simulink model "bici_v2"  (R2013a)
settings: Solver=ode3  SolverMode=SingleTasking  StartTime=0.0  StopTime=10.0  RelTol=1e-3
PreLoadFcn:
  | waijung.modelPreload; % Required for working with Waijung Blockset. Do not remove.
undefined symbols (not defined in the file or in its folder): HSEOSC, Link, LQFP176, ST, STM32F417IG
libraries: simulink x6, stm32f4_tim_lib x6, stm32f4_io_lib x2, stm32f4_adc_lib x1, stm32f4_device_config_lib x1
(part 2 of 2)

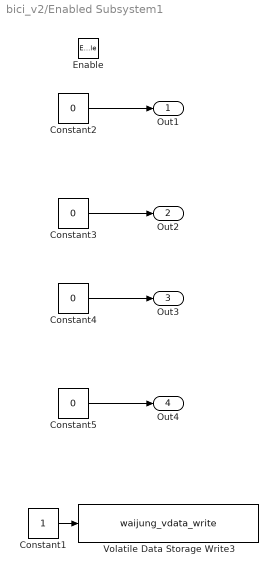
== system bici_v2/Enabled Subsystem1 ==
  Enable : EnablePort
  Constant1 : Constant
  Constant{2..5} (4 alike) : Constant  Value=0
  Volatile Data Storage Write3 : S-Function  FunctionName=waijung_vdata_write  Parameters=storagename,varname,sampletime,sampletimestr,blockid,storagetype,storagetypestr  EnableBusSupport=off  mask(waijung_vdata_write){storagename=c, varname=VolatileDataStorage3_c, sampletime=-1, sampletimestr=0.01, blockid=EnabledSubsystem1VolatileDataStorageWrite3, storagetype=double, storagetypestr=double}
      mask prompts: storagename "Storage Name"; varname "Variable name"; sampletime "Sample time (sec)"; sampletimestr "Compiled sample time (sec) in string"; storagetype "Data type"; storagetypestr "Data type string"
      mask help: This block implements write data to a buffer.
      mask init:
      | waijung_vdata_write_callback('init');
      mask Help: web(fullfile(waijungdocroot,'Volatile_Data_Storage_Write.htm'))
      mask TypeOptions storagename: condicion | c
      mask Callback storagename: waijung_vdata_write_callback('storagename');
      mask Callback varname: waijung_vdata_write_callback('varname');
      mask Callback sampletime: waijung_vdata_write_callback('sampletime');
      mask Callback sampletimestr: waijung_vdata_write_callback('sampletimestr');
      mask Callback blockid: waijung_vdata_write_callback('blockid');
      mask Callback storagetype: waijung_vdata_write_callback('storagetype');
      mask Display: text(0.95, 0.5, 'Buffer: c','ver','middle','hor','right');port_label('input',1,'D1(double)')
  Out1 : Outport
  Out2 : Outport  Port=2
  Out3 : Outport  Port=3
  Out4 : Outport  Port=4
  wires:
  Constant2/1 -> Out1/1
  Constant3/1 -> Out2/1
  Constant1/1 -> Volatile Data Storage Write3/1
  Constant4/1 -> Out3/1
  Constant5/1 -> Out4/1

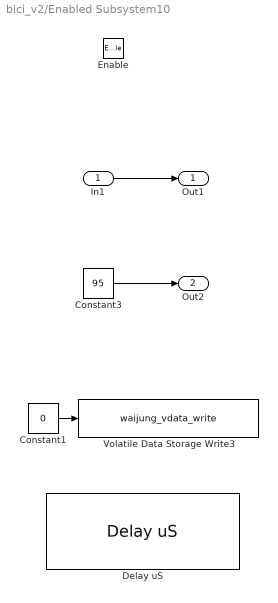
== system bici_v2/Enabled Subsystem10 ==
  In1 : Inport
  Enable : EnablePort
  Constant1 : Constant  Value=0
  Constant3 : Constant  Value=95
  Delay uS : stm32f4_tim_lib/Delay uS  delaytime=1  enableinput=off  enableoutput=off  inputtypearray=[0]  outputtypearray=[0]  sampletime=-1  sampletimestr=0.01  blockid=EnabledSubsystem10DelayuS
  Volatile Data Storage Write3 : S-Function  FunctionName=waijung_vdata_write  Parameters=storagename,varname,sampletime,sampletimestr,blockid,storagetype,storagetypestr  EnableBusSupport=off  mask(waijung_vdata_write){storagename=c, varname=VolatileDataStorage3_c, sampletime=-1, sampletimestr=0.01, blockid=EnabledSubsystem10VolatileDataStorageWrite3, storagetype=double, storagetypestr=double}
      mask prompts: storagename "Storage Name"; varname "Variable name"; sampletime "Sample time (sec)"; sampletimestr "Compiled sample time (sec) in string"; storagetype "Data type"; storagetypestr "Data type string"
      mask help: This block implements write data to a buffer.
      mask init:
      | waijung_vdata_write_callback('init');
      mask Help: web(fullfile(waijungdocroot,'Volatile_Data_Storage_Write.htm'))
      mask TypeOptions storagename: condicion | c
      mask Callback storagename: waijung_vdata_write_callback('storagename');
      mask Callback varname: waijung_vdata_write_callback('varname');
      mask Callback sampletime: waijung_vdata_write_callback('sampletime');
      mask Callback sampletimestr: waijung_vdata_write_callback('sampletimestr');
      mask Callback blockid: waijung_vdata_write_callback('blockid');
      mask Callback storagetype: waijung_vdata_write_callback('storagetype');
      mask Display: text(0.95, 0.5, 'Buffer: c','ver','middle','hor','right');port_label('input',1,'D1(double)')
  Out1 : Outport
  Out2 : Outport  Port=2
  wires:
  Constant3/1 -> Out2/1
  Constant1/1 -> Volatile Data Storage Write3/1
  In1/1 -> Out1/1

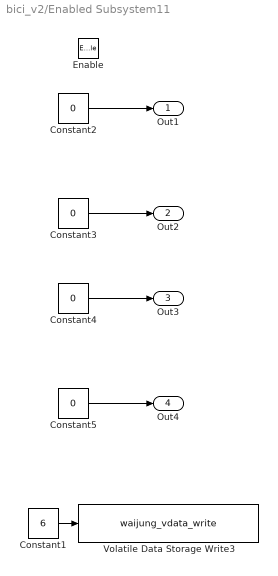
== system bici_v2/Enabled Subsystem11 ==
  Enable : EnablePort
  Constant1 : Constant  Value=6
  Constant{2..5} (4 alike) : Constant  Value=0
  Volatile Data Storage Write3 : S-Function  FunctionName=waijung_vdata_write  Parameters=storagename,varname,sampletime,sampletimestr,blockid,storagetype,storagetypestr  EnableBusSupport=off  mask(waijung_vdata_write){storagename=c, varname=VolatileDataStorage3_c, sampletime=-1, sampletimestr=0.01, blockid=EnabledSubsystem11VolatileDataStorageWrite3, storagetype=double, storagetypestr=double}
      mask prompts: storagename "Storage Name"; varname "Variable name"; sampletime "Sample time (sec)"; sampletimestr "Compiled sample time (sec) in string"; storagetype "Data type"; storagetypestr "Data type string"
      mask help: This block implements write data to a buffer.
      mask init:
      | waijung_vdata_write_callback('init');
      mask Help: web(fullfile(waijungdocroot,'Volatile_Data_Storage_Write.htm'))
      mask TypeOptions storagename: condicion | c
      mask Callback storagename: waijung_vdata_write_callback('storagename');
      mask Callback varname: waijung_vdata_write_callback('varname');
      mask Callback sampletime: waijung_vdata_write_callback('sampletime');
      mask Callback sampletimestr: waijung_vdata_write_callback('sampletimestr');
      mask Callback blockid: waijung_vdata_write_callback('blockid');
      mask Callback storagetype: waijung_vdata_write_callback('storagetype');
      mask Display: text(0.95, 0.5, 'Buffer: c','ver','middle','hor','right');port_label('input',1,'D1(double)')
  Out1 : Outport
  Out2 : Outport  Port=2
  Out3 : Outport  Port=3
  Out4 : Outport  Port=4
  wires:
  Constant2/1 -> Out1/1
  Constant3/1 -> Out2/1
  Constant1/1 -> Volatile Data Storage Write3/1
  Constant4/1 -> Out3/1
  Constant5/1 -> Out4/1

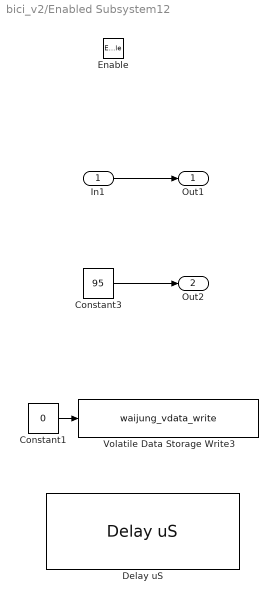
== system bici_v2/Enabled Subsystem12 ==
  In1 : Inport
  Enable : EnablePort
  Constant1 : Constant  Value=0
  Constant3 : Constant  Value=95
  Delay uS : stm32f4_tim_lib/Delay uS  delaytime=1  enableinput=off  enableoutput=off  inputtypearray=[0]  outputtypearray=[0]  sampletime=-1  sampletimestr=0.01  blockid=EnabledSubsystem12DelayuS
  Volatile Data Storage Write3 : S-Function  FunctionName=waijung_vdata_write  Parameters=storagename,varname,sampletime,sampletimestr,blockid,storagetype,storagetypestr  EnableBusSupport=off  mask(waijung_vdata_write){storagename=c, varname=VolatileDataStorage3_c, sampletime=-1, sampletimestr=0.01, blockid=EnabledSubsystem12VolatileDataStorageWrite3, storagetype=double, storagetypestr=double}
      mask prompts: storagename "Storage Name"; varname "Variable name"; sampletime "Sample time (sec)"; sampletimestr "Compiled sample time (sec) in string"; storagetype "Data type"; storagetypestr "Data type string"
      mask help: This block implements write data to a buffer.
      mask init:
      | waijung_vdata_write_callback('init');
      mask Help: web(fullfile(waijungdocroot,'Volatile_Data_Storage_Write.htm'))
      mask TypeOptions storagename: condicion | c
      mask Callback storagename: waijung_vdata_write_callback('storagename');
      mask Callback varname: waijung_vdata_write_callback('varname');
      mask Callback sampletime: waijung_vdata_write_callback('sampletime');
      mask Callback sampletimestr: waijung_vdata_write_callback('sampletimestr');
      mask Callback blockid: waijung_vdata_write_callback('blockid');
      mask Callback storagetype: waijung_vdata_write_callback('storagetype');
      mask Display: text(0.95, 0.5, 'Buffer: c','ver','middle','hor','right');port_label('input',1,'D1(double)')
  Out1 : Outport
  Out2 : Outport  Port=2
  wires:
  Constant3/1 -> Out2/1
  Constant1/1 -> Volatile Data Storage Write3/1
  In1/1 -> Out1/1

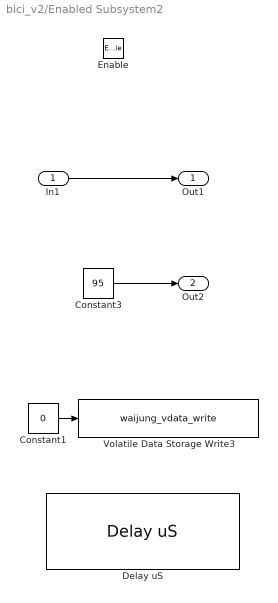
== system bici_v2/Enabled Subsystem2 ==
  In1 : Inport
  Enable : EnablePort
  Constant1 : Constant  Value=0
  Constant3 : Constant  Value=95
  Delay uS : stm32f4_tim_lib/Delay uS  delaytime=1  enableinput=off  enableoutput=off  inputtypearray=[0]  outputtypearray=[0]  sampletime=-1  sampletimestr=0.01  blockid=EnabledSubsystem2DelayuS
  Volatile Data Storage Write3 : S-Function  FunctionName=waijung_vdata_write  Parameters=storagename,varname,sampletime,sampletimestr,blockid,storagetype,storagetypestr  EnableBusSupport=off  mask(waijung_vdata_write){storagename=c, varname=VolatileDataStorage3_c, sampletime=-1, sampletimestr=0.01, blockid=EnabledSubsystem2VolatileDataStorageWrite3, storagetype=double, storagetypestr=double}
      mask prompts: storagename "Storage Name"; varname "Variable name"; sampletime "Sample time (sec)"; sampletimestr "Compiled sample time (sec) in string"; storagetype "Data type"; storagetypestr "Data type string"
      mask help: This block implements write data to a buffer.
      mask init:
      | waijung_vdata_write_callback('init');
      mask Help: web(fullfile(waijungdocroot,'Volatile_Data_Storage_Write.htm'))
      mask TypeOptions storagename: condicion | c
      mask Callback storagename: waijung_vdata_write_callback('storagename');
      mask Callback varname: waijung_vdata_write_callback('varname');
      mask Callback sampletime: waijung_vdata_write_callback('sampletime');
      mask Callback sampletimestr: waijung_vdata_write_callback('sampletimestr');
      mask Callback blockid: waijung_vdata_write_callback('blockid');
      mask Callback storagetype: waijung_vdata_write_callback('storagetype');
      mask Display: text(0.95, 0.5, 'Buffer: c','ver','middle','hor','right');port_label('input',1,'D1(double)')
  Out1 : Outport
  Out2 : Outport  Port=2
  wires:
  Constant3/1 -> Out2/1
  Constant1/1 -> Volatile Data Storage Write3/1
  In1/1 -> Out1/1

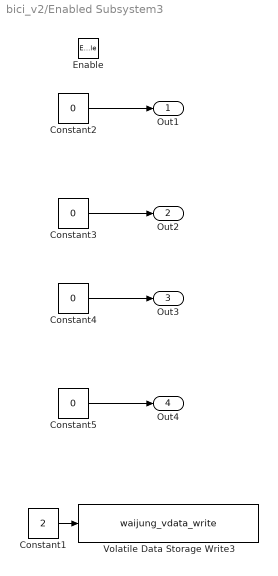
== system bici_v2/Enabled Subsystem3 ==
  Enable : EnablePort
  Constant1 : Constant  Value=2
  Constant{2..5} (4 alike) : Constant  Value=0
  Volatile Data Storage Write3 : S-Function  FunctionName=waijung_vdata_write  Parameters=storagename,varname,sampletime,sampletimestr,blockid,storagetype,storagetypestr  EnableBusSupport=off  mask(waijung_vdata_write){storagename=c, varname=VolatileDataStorage3_c, sampletime=-1, sampletimestr=0.01, blockid=EnabledSubsystem3VolatileDataStorageWrite3, storagetype=double, storagetypestr=double}
      mask prompts: storagename "Storage Name"; varname "Variable name"; sampletime "Sample time (sec)"; sampletimestr "Compiled sample time (sec) in string"; storagetype "Data type"; storagetypestr "Data type string"
      mask help: This block implements write data to a buffer.
      mask init:
      | waijung_vdata_write_callback('init');
      mask Help: web(fullfile(waijungdocroot,'Volatile_Data_Storage_Write.htm'))
      mask TypeOptions storagename: condicion | c
      mask Callback storagename: waijung_vdata_write_callback('storagename');
      mask Callback varname: waijung_vdata_write_callback('varname');
      mask Callback sampletime: waijung_vdata_write_callback('sampletime');
      mask Callback sampletimestr: waijung_vdata_write_callback('sampletimestr');
      mask Callback blockid: waijung_vdata_write_callback('blockid');
      mask Callback storagetype: waijung_vdata_write_callback('storagetype');
      mask Display: text(0.95, 0.5, 'Buffer: c','ver','middle','hor','right');port_label('input',1,'D1(double)')
  Out1 : Outport
  Out2 : Outport  Port=2
  Out3 : Outport  Port=3
  Out4 : Outport  Port=4
  wires:
  Constant2/1 -> Out1/1
  Constant3/1 -> Out2/1
  Constant1/1 -> Volatile Data Storage Write3/1
  Constant4/1 -> Out3/1
  Constant5/1 -> Out4/1

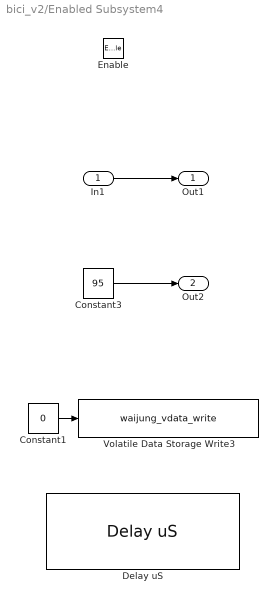
== system bici_v2/Enabled Subsystem4 ==
  In1 : Inport
  Enable : EnablePort
  Constant1 : Constant  Value=0
  Constant3 : Constant  Value=95
  Delay uS : stm32f4_tim_lib/Delay uS  delaytime=1  enableinput=off  enableoutput=off  inputtypearray=[0]  outputtypearray=[0]  sampletime=-1  sampletimestr=0.01  blockid=EnabledSubsystem4DelayuS
  Volatile Data Storage Write3 : S-Function  FunctionName=waijung_vdata_write  Parameters=storagename,varname,sampletime,sampletimestr,blockid,storagetype,storagetypestr  EnableBusSupport=off  mask(waijung_vdata_write){storagename=c, varname=VolatileDataStorage3_c, sampletime=-1, sampletimestr=0.01, blockid=EnabledSubsystem4VolatileDataStorageWrite3, storagetype=double, storagetypestr=double}
      mask prompts: storagename "Storage Name"; varname "Variable name"; sampletime "Sample time (sec)"; sampletimestr "Compiled sample time (sec) in string"; storagetype "Data type"; storagetypestr "Data type string"
      mask help: This block implements write data to a buffer.
      mask init:
      | waijung_vdata_write_callback('init');
      mask Help: web(fullfile(waijungdocroot,'Volatile_Data_Storage_Write.htm'))
      mask TypeOptions storagename: condicion | c
      mask Callback storagename: waijung_vdata_write_callback('storagename');
      mask Callback varname: waijung_vdata_write_callback('varname');
      mask Callback sampletime: waijung_vdata_write_callback('sampletime');
      mask Callback sampletimestr: waijung_vdata_write_callback('sampletimestr');
      mask Callback blockid: waijung_vdata_write_callback('blockid');
      mask Callback storagetype: waijung_vdata_write_callback('storagetype');
      mask Display: text(0.95, 0.5, 'Buffer: c','ver','middle','hor','right');port_label('input',1,'D1(double)')
  Out1 : Outport
  Out2 : Outport  Port=2
  wires:
  Constant3/1 -> Out2/1
  Constant1/1 -> Volatile Data Storage Write3/1
  In1/1 -> Out1/1

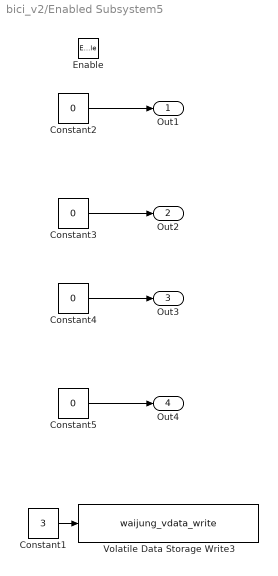
== system bici_v2/Enabled Subsystem5 ==
  Enable : EnablePort
  Constant1 : Constant  Value=3
  Constant{2..5} (4 alike) : Constant  Value=0
  Volatile Data Storage Write3 : S-Function  FunctionName=waijung_vdata_write  Parameters=storagename,varname,sampletime,sampletimestr,blockid,storagetype,storagetypestr  EnableBusSupport=off  mask(waijung_vdata_write){storagename=c, varname=VolatileDataStorage3_c, sampletime=-1, sampletimestr=0.01, blockid=EnabledSubsystem5VolatileDataStorageWrite3, storagetype=double, storagetypestr=double}
      mask prompts: storagename "Storage Name"; varname "Variable name"; sampletime "Sample time (sec)"; sampletimestr "Compiled sample time (sec) in string"; storagetype "Data type"; storagetypestr "Data type string"
      mask help: This block implements write data to a buffer.
      mask init:
      | waijung_vdata_write_callback('init');
      mask Help: web(fullfile(waijungdocroot,'Volatile_Data_Storage_Write.htm'))
      mask TypeOptions storagename: condicion | c
      mask Callback storagename: waijung_vdata_write_callback('storagename');
      mask Callback varname: waijung_vdata_write_callback('varname');
      mask Callback sampletime: waijung_vdata_write_callback('sampletime');
      mask Callback sampletimestr: waijung_vdata_write_callback('sampletimestr');
      mask Callback blockid: waijung_vdata_write_callback('blockid');
      mask Callback storagetype: waijung_vdata_write_callback('storagetype');
      mask Display: text(0.95, 0.5, 'Buffer: c','ver','middle','hor','right');port_label('input',1,'D1(double)')
  Out1 : Outport
  Out2 : Outport  Port=2
  Out3 : Outport  Port=3
  Out4 : Outport  Port=4
  wires:
  Constant2/1 -> Out1/1
  Constant3/1 -> Out2/1
  Constant1/1 -> Volatile Data Storage Write3/1
  Constant4/1 -> Out3/1
  Constant5/1 -> Out4/1

== system bici_v2/Enabled Subsystem6 ==
  In1 : Inport
  Enable : EnablePort
  Constant1 : Constant  Value=0
  Constant3 : Constant  Value=95
  Delay uS : stm32f4_tim_lib/Delay uS  delaytime=1  enableinput=off  enableoutput=off  inputtypearray=[0]  outputtypearray=[0]  sampletime=-1  sampletimestr=0.01  blockid=EnabledSubsystem6DelayuS
  Volatile Data Storage Write3 : S-Function  FunctionName=waijung_vdata_write  Parameters=storagename,varname,sampletime,sampletimestr,blockid,storagetype,storagetypestr  EnableBusSupport=off  mask(waijung_vdata_write){storagename=c, varname=VolatileDataStorage3_c, sampletime=-1, sampletimestr=0.01, blockid=EnabledSubsystem6VolatileDataStorageWrite3, storagetype=double, storagetypestr=double}
      mask prompts: storagename "Storage Name"; varname "Variable name"; sampletime "Sample time (sec)"; sampletimestr "Compiled sample time (sec) in string"; storagetype "Data type"; storagetypestr "Data type string"
      mask help: This block implements write data to a buffer.
      mask init:
      | waijung_vdata_write_callback('init');
      mask Help: web(fullfile(waijungdocroot,'Volatile_Data_Storage_Write.htm'))
      mask TypeOptions storagename: condicion | c
      mask Callback storagename: waijung_vdata_write_callback('storagename');
      mask Callback varname: waijung_vdata_write_callback('varname');
      mask Callback sampletime: waijung_vdata_write_callback('sampletime');
      mask Callback sampletimestr: waijung_vdata_write_callback('sampletimestr');
      mask Callback blockid: waijung_vdata_write_callback('blockid');
      mask Callback storagetype: waijung_vdata_write_callback('storagetype');
      mask Display: text(0.95, 0.5, 'Buffer: c','ver','middle','hor','right');port_label('input',1,'D1(double)')
  Out1 : Outport
  Out2 : Outport  Port=2
  wires:
  Constant3/1 -> Out2/1
  Constant1/1 -> Volatile Data Storage Write3/1
  In1/1 -> Out1/1

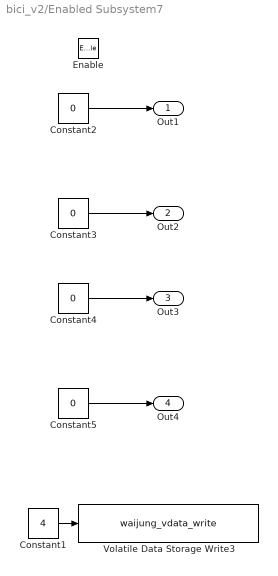
== system bici_v2/Enabled Subsystem7 ==
  Enable : EnablePort
  Constant1 : Constant  Value=4
  Constant{2..5} (4 alike) : Constant  Value=0
  Volatile Data Storage Write3 : S-Function  FunctionName=waijung_vdata_write  Parameters=storagename,varname,sampletime,sampletimestr,blockid,storagetype,storagetypestr  EnableBusSupport=off  mask(waijung_vdata_write){storagename=c, varname=VolatileDataStorage3_c, sampletime=-1, sampletimestr=0.01, blockid=EnabledSubsystem7VolatileDataStorageWrite3, storagetype=double, storagetypestr=double}
      mask prompts: storagename "Storage Name"; varname "Variable name"; sampletime "Sample time (sec)"; sampletimestr "Compiled sample time (sec) in string"; storagetype "Data type"; storagetypestr "Data type string"
      mask help: This block implements write data to a buffer.
      mask init:
      | waijung_vdata_write_callback('init');
      mask Help: web(fullfile(waijungdocroot,'Volatile_Data_Storage_Write.htm'))
      mask TypeOptions storagename: condicion | c
      mask Callback storagename: waijung_vdata_write_callback('storagename');
      mask Callback varname: waijung_vdata_write_callback('varname');
      mask Callback sampletime: waijung_vdata_write_callback('sampletime');
      mask Callback sampletimestr: waijung_vdata_write_callback('sampletimestr');
      mask Callback blockid: waijung_vdata_write_callback('blockid');
      mask Callback storagetype: waijung_vdata_write_callback('storagetype');
      mask Display: text(0.95, 0.5, 'Buffer: c','ver','middle','hor','right');port_label('input',1,'D1(double)')
  Out1 : Outport
  Out2 : Outport  Port=2
  Out3 : Outport  Port=3
  Out4 : Outport  Port=4
  wires:
  Constant2/1 -> Out1/1
  Constant3/1 -> Out2/1
  Constant1/1 -> Volatile Data Storage Write3/1
  Constant4/1 -> Out3/1
  Constant5/1 -> Out4/1

== system bici_v2/Enabled Subsystem8 ==
  In1 : Inport
  Enable : EnablePort
  Constant1 : Constant  Value=0
  Constant3 : Constant  Value=95
  Delay uS : stm32f4_tim_lib/Delay uS  delaytime=1  enableinput=off  enableoutput=off  inputtypearray=[0]  outputtypearray=[0]  sampletime=-1  sampletimestr=0.01  blockid=EnabledSubsystem8DelayuS
  Volatile Data Storage Write3 : S-Function  FunctionName=waijung_vdata_write  Parameters=storagename,varname,sampletime,sampletimestr,blockid,storagetype,storagetypestr  EnableBusSupport=off  mask(waijung_vdata_write){storagename=c, varname=VolatileDataStorage3_c, sampletime=-1, sampletimestr=0.01, blockid=EnabledSubsystem8VolatileDataStorageWrite3, storagetype=double, storagetypestr=double}
      mask prompts: storagename "Storage Name"; varname "Variable name"; sampletime "Sample time (sec)"; sampletimestr "Compiled sample time (sec) in string"; storagetype "Data type"; storagetypestr "Data type string"
      mask help: This block implements write data to a buffer.
      mask init:
      | waijung_vdata_write_callback('init');
      mask Help: web(fullfile(waijungdocroot,'Volatile_Data_Storage_Write.htm'))
      mask TypeOptions storagename: condicion | c
      mask Callback storagename: waijung_vdata_write_callback('storagename');
      mask Callback varname: waijung_vdata_write_callback('varname');
      mask Callback sampletime: waijung_vdata_write_callback('sampletime');
      mask Callback sampletimestr: waijung_vdata_write_callback('sampletimestr');
      mask Callback blockid: waijung_vdata_write_callback('blockid');
      mask Callback storagetype: waijung_vdata_write_callback('storagetype');
      mask Display: text(0.95, 0.5, 'Buffer: c','ver','middle','hor','right');port_label('input',1,'D1(double)')
  Out1 : Outport
  Out2 : Outport  Port=2
  wires:
  Constant3/1 -> Out2/1
  Constant1/1 -> Volatile Data Storage Write3/1
  In1/1 -> Out1/1

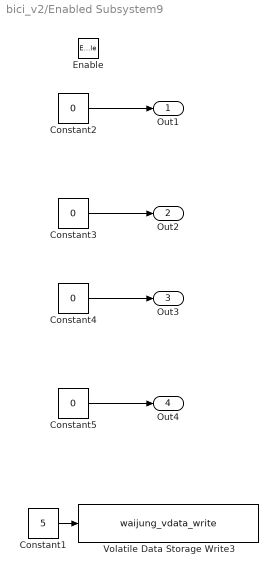
== system bici_v2/Enabled Subsystem9 ==
  Enable : EnablePort
  Constant1 : Constant  Value=5
  Constant{2..5} (4 alike) : Constant  Value=0
  Volatile Data Storage Write3 : S-Function  FunctionName=waijung_vdata_write  Parameters=storagename,varname,sampletime,sampletimestr,blockid,storagetype,storagetypestr  EnableBusSupport=off  mask(waijung_vdata_write){storagename=c, varname=VolatileDataStorage3_c, sampletime=-1, sampletimestr=0.01, blockid=EnabledSubsystem9VolatileDataStorageWrite3, storagetype=double, storagetypestr=double}
      mask prompts: storagename "Storage Name"; varname "Variable name"; sampletime "Sample time (sec)"; sampletimestr "Compiled sample time (sec) in string"; storagetype "Data type"; storagetypestr "Data type string"
      mask help: This block implements write data to a buffer.
      mask init:
      | waijung_vdata_write_callback('init');
      mask Help: web(fullfile(waijungdocroot,'Volatile_Data_Storage_Write.htm'))
      mask TypeOptions storagename: condicion | c
      mask Callback storagename: waijung_vdata_write_callback('storagename');
      mask Callback varname: waijung_vdata_write_callback('varname');
      mask Callback sampletime: waijung_vdata_write_callback('sampletime');
      mask Callback sampletimestr: waijung_vdata_write_callback('sampletimestr');
      mask Callback blockid: waijung_vdata_write_callback('blockid');
      mask Callback storagetype: waijung_vdata_write_callback('storagetype');
      mask Display: text(0.95, 0.5, 'Buffer: c','ver','middle','hor','right');port_label('input',1,'D1(double)')
  Out1 : Outport
  Out2 : Outport  Port=2
  Out3 : Outport  Port=3
  Out4 : Outport  Port=4
  wires:
  Constant2/1 -> Out1/1
  Constant3/1 -> Out2/1
  Constant1/1 -> Volatile Data Storage Write3/1
  Constant4/1 -> Out3/1
  Constant5/1 -> Out4/1

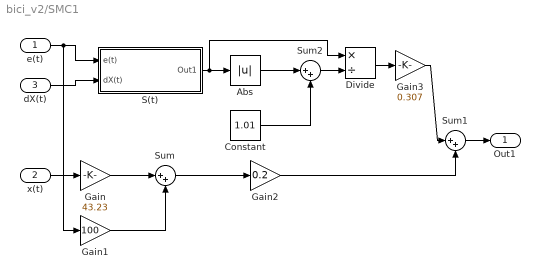
== system bici_v2/SMC1 ==
  e(t) : Inport
  x(t) : Inport  Port=2
  dX(t) : Inport  Port=3
  Abs : Abs
  Constant : Constant  Value=1.01
  Divide : Product  Inputs=*/
  Gain : Gain  Gain=43.23
  Gain1 : Gain  Gain=100
  Gain2 : Gain  Gain=0.2
  Gain3 : Gain  Gain=0.307
  S(t) : Subsystem  TreatAsAtomicUnit=on
  Sum : Sum  Inputs=|++
  Sum1 : Sum  Inputs=|++
  Sum2 : Sum  Inputs=|++
  Out1 : Outport
  wires:
  e(t)/1 -> Gain1/1, S(t)/1(e(t))
  dX(t)/1 -> S(t)/2(dX(t))
  x(t)/1 -> Gain/1
  Gain/1 -> Sum/1
  Gain1/1 -> Sum/2
  S(t)/1(Out1) -> Divide/1, Abs/1
  Abs/1 -> Sum2/1
  Constant/1 -> Sum2/2
  Sum2/1 -> Divide/2
  Divide/1 -> Gain3/1
  Gain3/1 -> Sum1/1
  Sum1/1 -> Out1/1
  Sum/1 -> Gain2/1
  Gain2/1 -> Sum1/2

== system bici_v2/SMC1/S(t) ==
  e(t) : Inport
  dX(t) : Inport  Port=2
  Gain : Gain  Gain=15
  Gain1 : Gain  Gain=100
  Gain2 : Gain  Gain=-1
  Integrator : Integrator  LimitOutput=on  UpperSaturationLimit=80  LowerSaturationLimit=0
  Sum : Sum  Inputs=|+++
  Out1 : Outport
  wires:
  Gain/1 -> Sum/1
  e(t)/1 -> Integrator/1, Gain/1
  Gain1/1 -> Sum/2
  Integrator/1 -> Gain1/1
  Sum/1 -> Out1/1
  dX(t)/1 -> Gain2/1
  Gain2/1 -> Sum/3
